simulink model "mavsim_chap4"  (Simulink 7.5)
settings: Solver=ode45  StartTime=0.0  StopTime=10000  RelTol=1e-3
undefined symbols (not defined in the file or in its folder): drawAircraft, forces_moments, P, plotmavstatevariables
libraries: simulink x4
settings Model: Creator=beard  LastModifiedBy=beard
settings OptimizationCC: InitFltsAndDblsToZero=on
settings DebuggingCC: StrictBusMsg=Warning

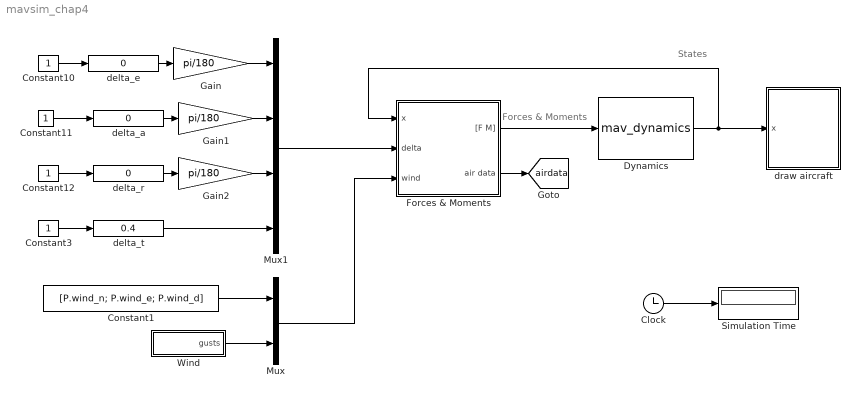
== system mavsim_chap4 ==
  note: Forces & Moments
  note: States
  Clock : Clock
      settings: Decimation=10
  Constant1 : Constant  Value=[P.wind_n; P.wind_e; P.wind_d]  OutDataType=sfix(16)  OutScaling=2^0
  Constant{3,10..12} (4 alike) : Constant  OutDataType=sfix(16)  OutScaling=2^0
  Dynamics : S-Function  FunctionName=mav_dynamics  Parameters=mass,Jx,Jy,Jz,Jxz,pn0,pe0,pd0,u0,v0,w0,phi0,theta0,psi0,p0,q0,r0  EnableBusSupport=off  mask{mass=P.mass, Jx=P.Jx, Jy=P.Jy, Jz=P.Jz, Jxz=P.Jxz, pn0=P.pn0, pe0=P.pe0, pd0=P.pd0, u0=P.u0, v0=P.v0, w0=P.w0, phi0=P.phi0, theta0=P.theta0, psi0=P.psi0, p0=P.p0, q0=P.q0, r0=P.r0}
      mask prompts: pn0 "Initial North position"; pe0 "Initial East position"; pd0 "Initial Down position"; u0 "Initial velocy u0"; v0 "Initial velocity v0"; w0 "Initial velocity w0"; phi0 "Initial roll angle"; theta0 "Initial pitch angle"; psi0 "Initial yaw angle"; p0 "Initial roll rate"; q0 "Initial pitch rate"; r0 "Initial yaw rate"
  Forces & Moments : Subsystem
  Gain : Gain  Gain=pi/180  ParameterDataType=fixdt(1, 16)  ParameterScaling=2^0  OutDataType=fixdt(1, 16)  OutScaling=2^0
  Gain1 : Gain  Gain=pi/180  ParameterDataType=fixdt(1, 16)  ParameterScaling=2^0  OutDataType=fixdt(1, 16)  OutScaling=2^0
  Gain2 : Gain  Gain=pi/180  ParameterDataType=fixdt(1, 16)  ParameterScaling=2^0  OutDataType=fixdt(1, 16)  OutScaling=2^0
  Mux : Mux  Inputs=2
  Mux1 : Mux
  Simulation Time : Display
  Wind : Subsystem
  delta_a : simulink/Math Operations/Slider Gain  SystemSampleTime=-1  low=-45  gain=0  high=45
  delta_e : simulink/Math Operations/Slider Gain  SystemSampleTime=-1  low=-45  gain=0  high=45
  delta_r : simulink/Math Operations/Slider Gain  SystemSampleTime=-1  low=-45  gain=0  high=45
  delta_t : simulink/Math Operations/Slider Gain  SystemSampleTime=-1  low=0  gain=0.4  high=1
  draw aircraft : Subsystem
      mask init:
      | % parameters for drawing aircraft
      |   % scale size
      |   size = 20;
      |   fuse_l1    = 7;
      |   fuse_l2    = 4;
      |   fuse_l3    = 15;
      |   fuse_w     = 2;
      |   wing_l     = 6;
      |   wing_w     = 20;
      |   tail_l     = 3;
      |   tail_h     = 3;
      |   tailwing_w = 10;
      |   tailwing_l = 3;
      |   % colors
      |   red     = [1, 0, 0];
      |   green   = [0, 1, 0];
      |   blue    = [0, 0, 1];
      |   yellow  = [1,1,0];
      |   magenta = [0, 1, 1];
      |   
      | 
      | % define vertices and faces for aircraft
      |   V = [...
      |     fuse_l1,             0,             0;...        % point 1
      |     fuse_l2,            -fuse_w/2,     -fuse_w/2;... % point 2     
      |     fuse_l2,             fuse_w/2,     -fuse_w/2;... % point 3     
      |     fuse_l2,             fuse_w/2,      fuse_w/2;... % point 4
      |     fuse_l2,            -fuse_w/2,      fuse_w/2;... % point 5
      |    -fuse_l3,             0,             0;...        % point 6
      |     0,                   wing_w/2,      0;...        % point 7
      |    -wing_l,              wing_w/2,      0;...        % point 8
      |    -wing_l,             -wing_w/2,      0;...        % point 9
      |     0,                  -wing_w/2,      0;...        % point 10
      |    -fuse_l3+tailwing_l,  tailwing_w/2,  0;...        % point 11
      |    -fuse_l3,             tailwing_w/2,  0;...        % point 12
      |    -fuse_l3,            -tailwing_w/2,  0;...        % point 13
      |    -fuse_l3+tailwing_l, -tailwing_w/2,  0;...        % point 14
      |    -fuse_l3+tailwing_l,  0,             0;...        % point 15
      |    -fuse_l3+tailwing_l,  0,             -tail_h;...  % point 16
      |    -fuse_l3,             0,             -tail_h;...  % point 17
      |   ];
      |   
      |   F = [...
      |         1,  2,  3,  1;... % nose-top
      |         1,  3,  4,  1;... % nose-left
      |         1,  4,  5,  1;... % nose-bottom
      |         1,  5,  2,  1;... % nose-right
      |         2,  3,  6,  2;... % fuselage-top
      |         3,  6,  4,  3;... % fuselage-left
      |         4,  6,  5,  4;... % fuselage-bottom
      |         2,  5,  6,  2;... % fuselage-right
      |         7,  8,  9, 10;... % wing
      |        11, 12, 13, 14;... % tailwing
      |         6, 15, 17, 17;... % tail
      |         
      |   ];  
      |   
      |   colors = [...
      |         yellow;... % nose-top
      |         yellow;... % nose-left
      |         yellow;... % nose-bottom
      |         yellow;... % nose-right
      |         blue;... % fuselage-top
      |         blue;... % fuselage-left
      |         red;... % fuselage-bottom
      |         blue;... % fuselage-right
      |         green;... % wing
      |         green;... % tailwing
      |         blue;... % tail
      |     ];
      | 
      |   V = size*V;   % rescale vertices
      mask Display: image(imread('tv.jpg'))
  tag scope: airdata=global
  wires:
  Constant10/1 -> delta_e/1
  Constant11/1 -> delta_a/1
  Constant12/1 -> delta_r/1
  Dynamics/1 -> Forces & Moments/1(x), draw aircraft/1(x)
  delta_r/1 -> Gain2/1
  delta_a/1 -> Gain1/1
  delta_e/1 -> Gain/1
  Constant3/1 -> delta_t/1
  delta_t/1 -> Mux1/4
  Mux1/1 -> Forces & Moments/2(delta)
  Forces & Moments/1("[F M]") -> Dynamics/1
  Clock/1 -> Simulation Time/1
  Mux/1 -> Forces & Moments/3(wind)
  Wind/1(gusts) -> Mux/2
  Constant1/1 -> Mux/1
  Forces & Moments/2(air data) -> [airdata]
  Gain/1 -> Mux1/1
  Gain1/1 -> Mux1/2
  Gain2/1 -> Mux1/3

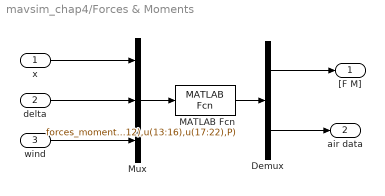
== system mavsim_chap4/Forces & Moments ==
  x : Inport
  delta : Inport  Port=2
  wind : Inport  Port=3
  Demux : Demux  Outputs=[6;6]
  MATLAB Fcn : MATLABFcn  MATLABFcn=forces_moments(u(1:12),u(13:16),u(17:22),P)  OutputDimensions=12
  Mux : Mux  Inputs=3
  "[F M]" : Outport
  air data : Outport  Port=2
  wires:
  x/1 -> Mux/1
  delta/1 -> Mux/2
  wind/1 -> Mux/3
  MATLAB Fcn/1 -> Demux/1
  Demux/1 -> "[F M]"/1
  Mux/1 -> MATLAB Fcn/1
  Demux/2 -> air data/1

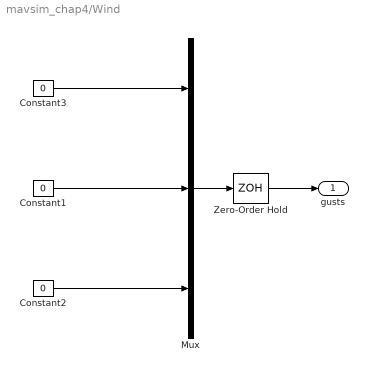
== system mavsim_chap4/Wind ==
  Constant1 : Constant  Value=0  OutDataType=sfix(16)  OutScaling=2^0
  Constant2 : Constant  Value=0  OutDataType=sfix(16)  OutScaling=2^0
  Constant3 : Constant  Value=0  OutDataType=sfix(16)  OutScaling=2^0
  Mux : Mux  Inputs=3
  Zero-Order Hold : ZeroOrderHold  SampleTime=P.Ts
  gusts : Outport
  wires:
  Constant3/1 -> Mux/1
  Constant1/1 -> Mux/2
  Constant2/1 -> Mux/3
  Mux/1 -> Zero-Order Hold/1
  Zero-Order Hold/1 -> gusts/1

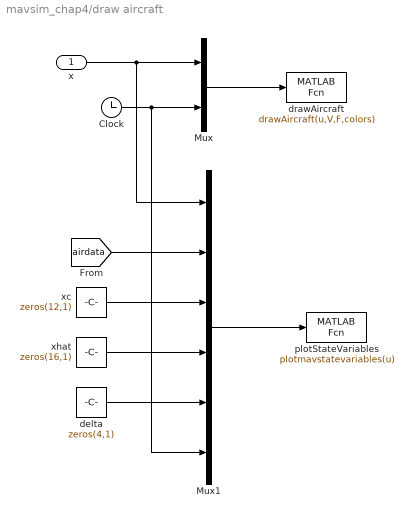
== system mavsim_chap4/draw aircraft ==
  x : Inport
  Clock : Clock
      settings: Decimation=10
  Mux : Mux  Inputs=2
  Mux1 : Mux  Inputs=6
  delta : Constant  Value=zeros(4,1)  OutDataType=sfix(16)  OutScaling=2^0
  drawAircraft : MATLABFcn  MATLABFcn=drawAircraft(u,V,F,colors)  OutputDimensions=0  SampleTime=0.1
  plotStateVariables : MATLABFcn  MATLABFcn=plotmavstatevariables(u)  OutputDimensions=0  SampleTime=0.1
  xc : Constant  Value=zeros(12,1)  OutDataType=sfix(16)  OutScaling=2^0
  xhat : Constant  Value=zeros(16,1)  OutDataType=sfix(16)  OutScaling=2^0
  wires:
  [airdata] -> Mux1/2
  delta/1 -> Mux1/5
  xc/1 -> Mux1/3
  xhat/1 -> Mux1/4
  Mux1/1 -> plotStateVariables/1
  Clock/1 -> Mux1/6, Mux/2
  x/1 -> Mux1/1, Mux/1
  Mux/1 -> drawAircraft/1
